simulink model "simulation"  (R2016a)
settings: Solver=VariableStepAuto  StartTime=0.0  StopTime=100  FixedStep=0.01  MaxStep=0.01  RelTol=1e-3
values from neighbouring files (symbols this model uses):
  A_2 = zeros(N)    [main.m]
  A_c_2 = [A_2 l_c'; zeros(1,N+1)]    [main.m]
  r_init = zeros(3,N)    [main.m]
  r_rel_1 = r_rel_cube    [create_r_relative.m]
  r_rel_2 = r_rel_cube    [create_r_relative.m]
  r_rel_3 = r_rel_cube    [create_r_relative.m]
  xi_init = zeros(6,N)    [main.m]
undefined symbols (not defined in the file or in its folder): A, A_c
libraries: simulink x2
settings Model: Creator=Jens  LastModifiedBy=Jens

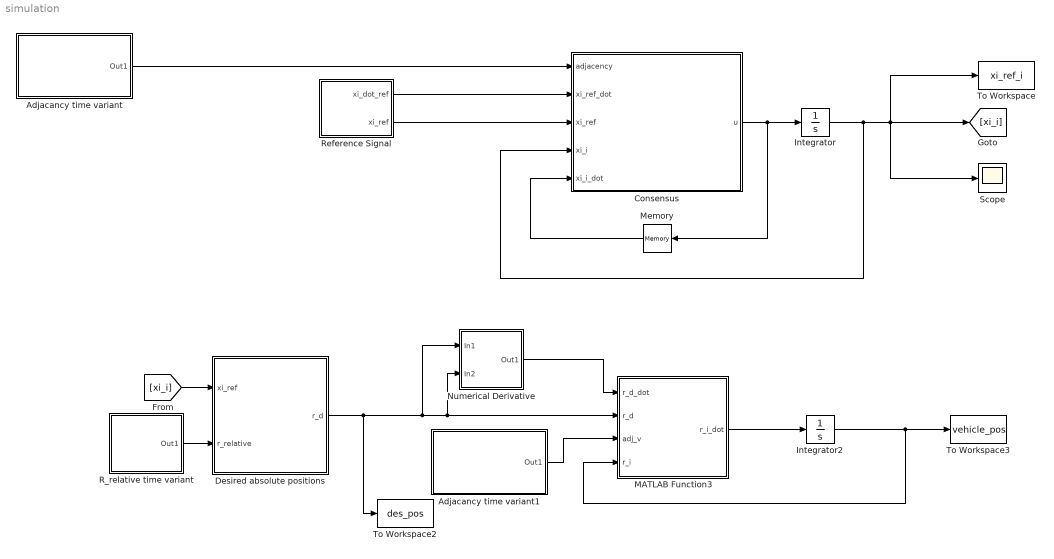
== system simulation ==
  Adjacancy time variant : Subsystem
  Adjacancy time variant1 : Subsystem
  Consensus : MATLAB Function  TreatAsAtomicUnit=on
      settings: MinAlgLoopOccurrences=on
  Desired absolute positions : MATLAB Function  TreatAsAtomicUnit=on
  Integrator : Integrator  InitialCondition=xi_init
  Integrator2 : Integrator  InitialCondition=r_init
  MATLAB Function3 : MATLAB Function  TreatAsAtomicUnit=on
  Memory : Memory
  Numerical Derivative : Subsystem
  R_relative time variant : Subsystem
  Reference Signal : Subsystem
  Scope : Scope
  To Workspace : ToWorkspace  VariableName=xi_ref_i  SaveFormat=Timeseries  SampleTime=-1
  To Workspace2 : ToWorkspace  VariableName=des_pos  SaveFormat=Timeseries  SampleTime=-1
  To Workspace3 : ToWorkspace  VariableName=vehicle_pos  SaveFormat=Timeseries  SampleTime=-1
  wires:
  Integrator/1 -> Scope/1, [xi_i], To Workspace/1, Consensus/4(xi_i)
  Consensus/1(u) -> Integrator/1, Memory/1
  Memory/1 -> Consensus/5(xi_i_dot)
  [xi_i] -> Desired absolute positions/1(xi_ref)
  Desired absolute positions/1(r_d) -> Numerical Derivative/1(In1), MATLAB Function3/2(r_d), Numerical Derivative/2(In2), To Workspace2/1
  Reference Signal/1(xi_dot_ref) -> Consensus/2(xi_ref_dot)
  Reference Signal/2(xi_ref) -> Consensus/3(xi_ref)
  MATLAB Function3/1(r_i_dot) -> Integrator2/1
  Integrator2/1 -> To Workspace3/1, MATLAB Function3/4(r_i)
  Numerical Derivative/1(Out1) -> MATLAB Function3/1(r_d_dot)
  Adjacancy time variant/1(Out1) -> Consensus/1(adjacency)
  R_relative time variant/1(Out1) -> Desired absolute positions/2(r_relative)
  Adjacancy time variant1/1(Out1) -> MATLAB Function3/3(adj_v)

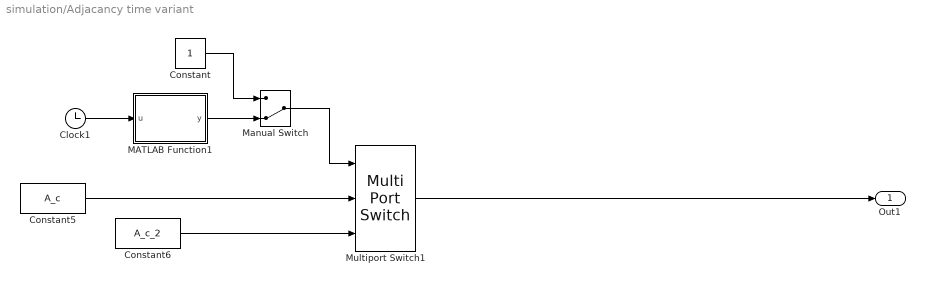
== system simulation/Adjacancy time variant ==
  Clock1 : Clock
  Constant : Constant
  Constant5 : Constant  Value=A_c
  Constant6 : Constant  Value=A_c_2
  MATLAB Function1 : MATLAB Function  TreatAsAtomicUnit=on
  Manual Switch : ManualSwitch  CurrentSetting=0
  Multiport Switch1 : MultiPortSwitch  Inputs=2
  Out1 : Outport
  wires:
  Manual Switch/1 -> Multiport Switch1/1
  Clock1/1 -> MATLAB Function1/1(u)
  Multiport Switch1/1 -> Out1/1
  Constant6/1 -> Multiport Switch1/3
  Constant5/1 -> Multiport Switch1/2
  Constant/1 -> Manual Switch/1
  MATLAB Function1/1(y) -> Manual Switch/2

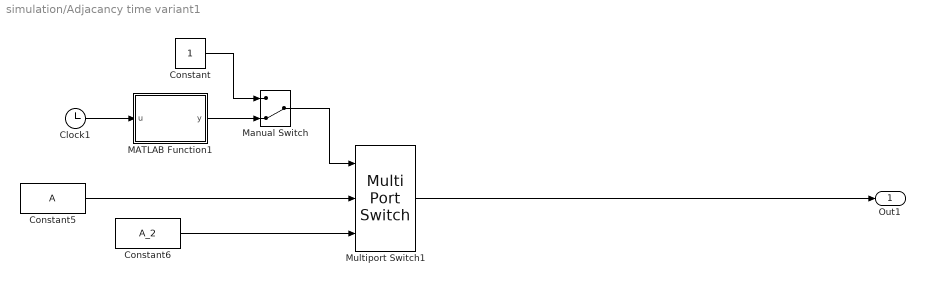
== system simulation/Adjacancy time variant1 ==
  Clock1 : Clock
  Constant : Constant
  Constant5 : Constant  Value=A
  Constant6 : Constant  Value=A_2
  MATLAB Function1 : MATLAB Function  TreatAsAtomicUnit=on
  Manual Switch : ManualSwitch  CurrentSetting=0
  Multiport Switch1 : MultiPortSwitch  Inputs=2
  Out1 : Outport
  wires:
  Manual Switch/1 -> Multiport Switch1/1
  Clock1/1 -> MATLAB Function1/1(u)
  Multiport Switch1/1 -> Out1/1
  Constant6/1 -> Multiport Switch1/3
  Constant5/1 -> Multiport Switch1/2
  Constant/1 -> Manual Switch/1
  MATLAB Function1/1(y) -> Manual Switch/2

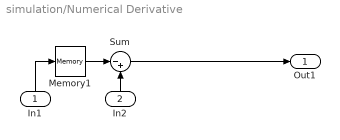
== system simulation/Numerical Derivative ==
  In1 : Inport
  In2 : Inport  Port=2
  Memory1 : Memory
  Sum : Sum  Inputs=|-+
  Out1 : Outport
  wires:
  In2/1 -> Sum/2
  In1/1 -> Memory1/1
  Memory1/1 -> Sum/1
  Sum/1 -> Out1/1

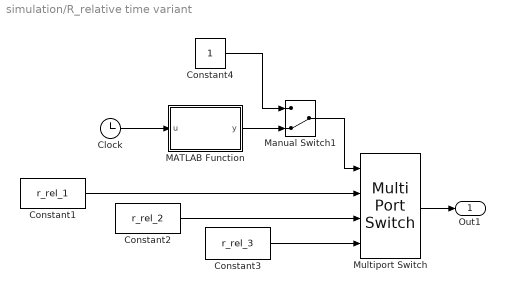
== system simulation/R_relative time variant ==
  Clock : Clock
  Constant1 : Constant  Value=r_rel_1
  Constant2 : Constant  Value=r_rel_2
  Constant3 : Constant  Value=r_rel_3
  Constant4 : Constant
  MATLAB Function : MATLAB Function  TreatAsAtomicUnit=on
  Manual Switch1 : ManualSwitch  CurrentSetting=0
  Multiport Switch : MultiPortSwitch
  Out1 : Outport
  wires:
  Constant4/1 -> Manual Switch1/1
  MATLAB Function/1(y) -> Manual Switch1/2
  Manual Switch1/1 -> Multiport Switch/1
  Constant1/1 -> Multiport Switch/2
  Constant2/1 -> Multiport Switch/3
  Clock/1 -> MATLAB Function/1(u)
  Multiport Switch/1 -> Out1/1
  Constant3/1 -> Multiport Switch/4

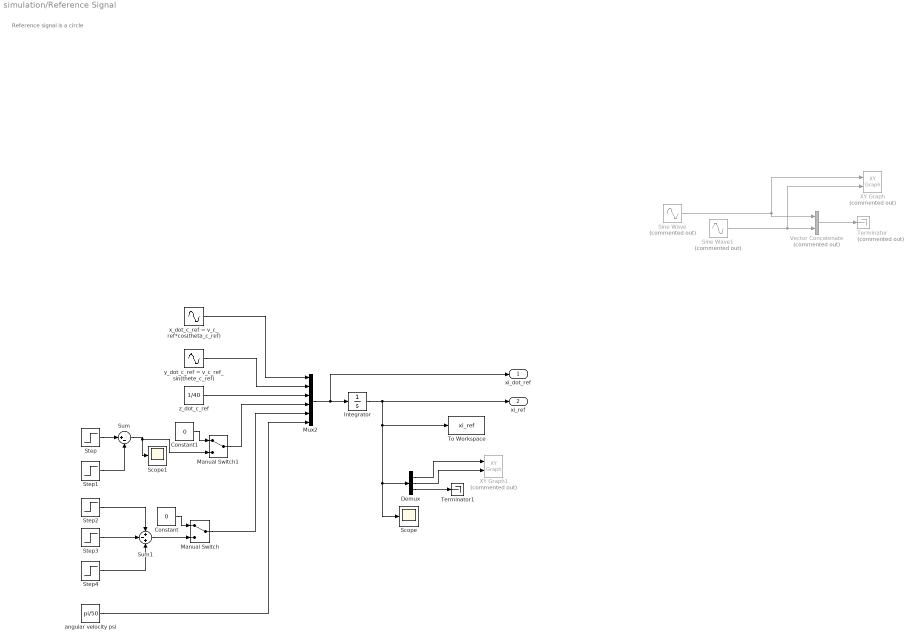
== system simulation/Reference Signal ==
  note: Reference signal is a circle
  Constant : Constant  Value=0
  Constant1 : Constant  Value=0
  Demux : Demux  Outputs=3
  Integrator : Integrator  InitialCondition=[0;0;0;0;0;0]
  Manual Switch : ManualSwitch
  Manual Switch1 : ManualSwitch
  Mux2 : Mux  Inputs=6
  Scope : Scope
  Scope1 : Scope
  Sine Wave : Sin  Commented=on  Phase=pi/2  SampleTime=0
  Sine Wave1 : Sin  Commented=on  SampleTime=0
  Step : Step  Time=20  After=pi/10  SampleTime=0
  Step1 : Step  Time=40  After=pi/10  SampleTime=0
  Step2 : Step  Time=10  After=pi/30  SampleTime=0
  Step3 : Step  Time=15  After=pi/30*2  SampleTime=0
  Step4 : Step  Time=20  After=pi/30  SampleTime=0
  Sum : Sum  Inputs=|+-
  Sum1 : Sum  Inputs=+-+
  Terminator : Terminator  Commented=on
  Terminator1 : Terminator
  To Workspace : ToWorkspace  VariableName=xi_ref  SaveFormat=Timeseries  SampleTime=-1
  Vector Concatenate : Concatenate  Commented=on
  XY Graph : simulink/Sinks/XY Graph  Commented=on  xmin=-1  xmax=1  ymin=-1  ymax=1  st=-1
  XY Graph1 : simulink/Sinks/XY Graph  Commented=on  xmin=-1  xmax=1  ymin=-1  ymax=3  st=-1
  angular velocity psi : Constant  Value=pi/50
  x_dot_c_ref = v_c_ref*cos(theta_c_ref) : Sin  Amplitude=9*pi/500  Frequency=pi/50  Phase=pi/2  SampleTime=0
  y_dot_c_ref = v_c_ref_sin(thete_c_ref) : Sin  Amplitude=9*pi/500  Frequency=pi/50  SampleTime=0
  z_dot_c_ref : Constant  Value=1/40
  xi_dot_ref : Outport
  xi_ref : Outport  Port=2
  wires:
  Sine Wave1/1 -> XY Graph/2, Vector Concatenate/2
  Sine Wave/1 -> Vector Concatenate/1, XY Graph/1
  Vector Concatenate/1 -> Terminator/1
  Demux/1 -> XY Graph1/1
  Demux/2 -> XY Graph1/2
  Demux/3 -> Terminator1/1
  y_dot_c_ref = v_c_ref_sin(thete_c_ref)/1 -> Mux2/2
  x_dot_c_ref = v_c_ref*cos(theta_c_ref)/1 -> Mux2/1
  Mux2/1 -> xi_dot_ref/1, Integrator/1
  Integrator/1 -> To Workspace/1, Scope/1, Demux/1, xi_ref/1
  angular velocity psi/1 -> Mux2/6
  z_dot_c_ref/1 -> Mux2/3
  Step/1 -> Sum/1
  Step1/1 -> Sum/2
  Step2/1 -> Sum1/1
  Step3/1 -> Sum1/2
  Step4/1 -> Sum1/3
  Sum1/1 -> Manual Switch/2
  Manual Switch/1 -> Mux2/5
  Constant/1 -> Manual Switch/1
  Sum/1 -> Manual Switch1/2, Scope1/1
  Constant1/1 -> Manual Switch1/1
  Manual Switch1/1 -> Mux2/4

== matlab function simulation/Adjacancy time variant/MATLAB Function1 ==
  data: u input; y output
function y = fcn(u)

if (u >= 20 && u < 60)
    y = 2;
else
    y = 1;
end

== matlab function simulation/Consensus ==
  data: adjacency input; u output; xi_ref_dot input; xi_ref input; xi_i input; xi_i_dot input
function u = fcn(adjacency, xi_ref_dot, xi_ref, xi_i, xi_i_dot)
% calculates u = xi_i_dot for all vehicles according to the conensus
% formula for time-varying reference state (access to the leader only to a subgroup)

% Number of vehicles
N = size(adjacency,1)-1;
% initialize output u to zero
u = zeros(6,N);

% scalar to influence convergence speed
gamma = 1;

% formula to calculate xi_dot_i = u_i for each vehicle compare p. 196
% [REN08] formula 10.1
% u consists of six states per vehicle in a 6xN matrix / updates each
% vehicle after another (6 states per iteration of outer for loop)
for i=1:1:N
    eta = sum(adjacency(i,:));
    % if vehicle has no incoming connection (equal to eta = 0) u is set to zero therefore the
    % information states don't change and remain constant
    if (eta == 0)
        u(:,i) = zeros(6,1);
    else
        temp = zeros(6,1);
        for j=1:1:N
            temp = temp + adjacency(i,j)*(xi_i_dot(:,j)-gamma*(xi_i(:,i)-xi_i(:,j)));
        end
        u(:,i) = 1/eta * temp + 1/eta * adjacency(i,N+1)*(xi_ref_dot-gamma*(xi_i(:,i)-xi_ref));
    end    
end

== matlab function simulation/R_relative time variant/MATLAB Function ==
  data: u input; y output
function y = fcn(u)

if (u < 20)
    y = 1;
elseif (u >= 20 && u < 50)
    y = 2;
elseif (u >= 50 && u < 100)
    y = 3;
else
    y = 1;
end

== matlab function simulation/Desired absolute positions ==
  data: xi_ref input; r_d output; r_relative input
function r_d  = desired_pos_abs(xi_ref, r_relative)
% desired_pos_abs computes the desired absolute positions depending on the
% reference frame and the relative coordinates of the desired positions
% outputs x_d and y_d in a vector r_d
% inputs are xi_ref = [x_coordinate_frame, y_coordinate_frame,
% theta_coordinate frame] the reference frame

r_d = zeros(size(r_relative));

psi = xi_ref(6);
phi = xi_ref(5);
theta = xi_ref(4);

% Drehmatrix Dz
Dz = [cos(psi) -sin(psi) 0
      sin(psi)  cos(psi) 0
         0          0    1];

% Drehmatrix Dy    
Dy = [cos(phi)  0   sin(phi)
         0      1      0
     -sin(phi)  0   cos(phi)];

% Drehmatrix Dx
Dx = [1     0         0          
      0  cos(theta) -sin(theta)
      0  sin(theta)  cos(theta)];
  
  for i=1:1:size(r_relative,2)
      r_d(:,i) = xi_ref(1:3)' + Dz*Dy*Dx*r_relative(:,i);
  end

end

== matlab function simulation/MATLAB Function3 ==
  data: r_d_dot input; r_d input; adj_v input; r_i_dot output; r_i input
function r_i_dot = fcn(r_d_dot, r_d, adj_v, r_i)

N = size(adj_v,1);
u = zeros(3,N);
alpha = 1;
temp = zeros(3,1);

for i=1:1:N
    for j=1:1:N
        temp = temp + adj_v(i,j)*((r_i(:,i)-r_d(:,i))-(r_i(:,j)-r_d(:,j)));
    end
    u(:,i) = r_d_dot(:,i)-alpha*(r_i(:,i)-r_d(:,i)) - temp;
    temp = zeros(3,1);
end

r_i_dot = u;

== matlab function simulation/Adjacancy time variant1/MATLAB Function1 ==
  data: u input; y output
function y = fcn(u)

if (u >= 20 && u < 60)
    y = 2;
else
    y = 1;
end
